simulink model "imugetmeas"  (R2025a)
settings: Solver=VariableStepAuto  StartTime=0.0  StopTime=10.0  RelTol=1e-3
undefined symbols (not defined in the file or in its folder): axang2rotm, fractalcoef
libraries: mspsensorlib x2
settings Model: Creator=nicolls  LastModifiedBy=nicolls

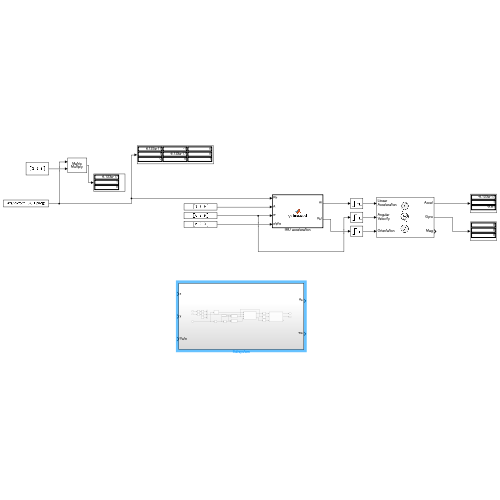
[thumbnail: Simulink's stored preview of the top-level diagram]
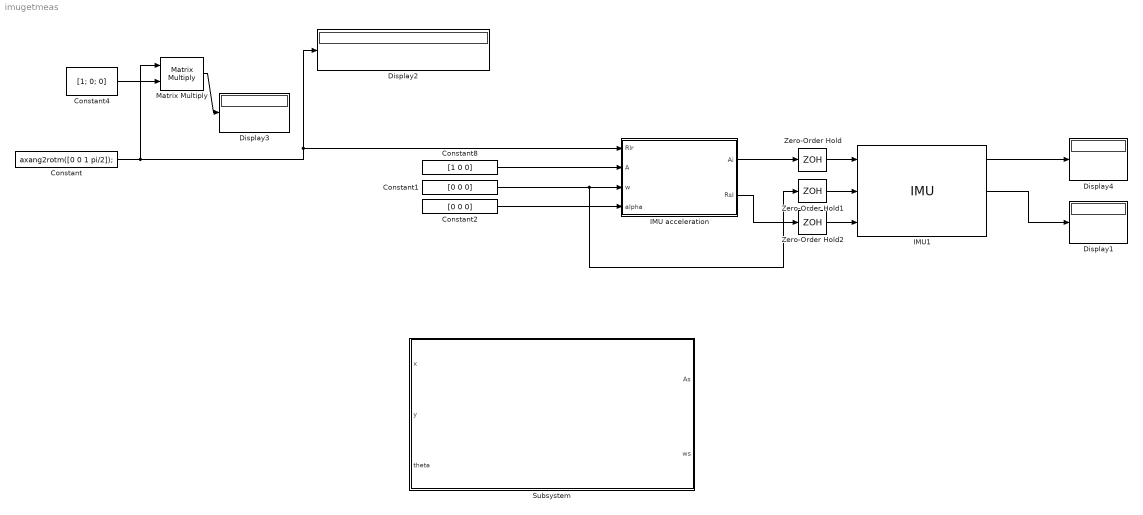
== system imugetmeas ==
  Constant : Constant  Value=axang2rotm([0 0 1 pi/2]);
  Constant1 : Constant  Value=[0 0 0]  VectorParams1D=off
  Constant2 : Constant  Value=[0 0 0]  VectorParams1D=off
  Constant4 : Constant  Value=[1; 0; 0]
  Constant8 : Constant  Value=[1 0 0]  VectorParams1D=off
  Display{1..4} (4 alike) : Display
  IMU acceleration : MATLAB Function  TreatAsAtomicUnit=on
  IMU1 : mspsensorlib/IMU  DispRefFrame=ENU  TemperaturePort=off  Temperature=25  MagneticFieldPort=off  MagneticFieldNED=[ 27.5550, -2.4169, -16.0849 ]  MagneticFieldENU=[ -2.4169, 27.5550, 16.0849 ]  SeedDouble=67  SimulateUsing=Interpreted execution  AccelParamsMeasurementRange=Inf  AccelParamsResolution=0  AccelParamsConstantBias=[ 0, 0, 0 ]  AccelParamsAxesMisalignment=[ 100, 0, 0; 0, 100, 0; 0, 0, 100 ]  AccelParamsNoiseDensity=[ 0, 0, 0 ]  AccelParamsBiasInstability=[ 0, 0, 0 ]  AccelParamsBiasInstabilityNumerator=fractalcoef().Numerator  AccelParamsBiasInstabilityDenominator=fractalcoef().Denominator  AccelParamsRandomWalk=[ 0, 0, 0 ]  AccelParamsNoiseType=double-sided  AccelParamsTemperatureBias=[ 0, 0, 0 ]  AccelParamsTemperatureScaleFactor=[ 0, 0, 0 ]  GyroParamsMeasurementRange=Inf  GyroParamsResolution=0  GyroParamsConstantBias=[ 0, 0, 0 ]  GyroParamsAxesMisalignment=[ 100, 0, 0; 0, 100, 0; 0, 0, 100 ]  GyroParamsAccelerationBias=[ 0, 0, 0 ]  GyroParamsNoiseDensity=[ 0, 0, 0 ]  GyroParamsBiasInstability=[ 0, 0, 0 ]  GyroParamsBiasInstabilityNumerator=fractalcoef().Numerator  GyroParamsBiasInstabilityDenominator=fractalcoef().Denominator  GyroParamsRandomWalk=[ 0, 0, 0 ]  GyroParamsNoiseType=double-sided  GyroParamsTemperatureBias=[ 0, 0, 0 ]  GyroParamsTemperatureScaleFactor=[ 0, 0, 0 ]  MagParamsMeasurementRange=Inf  MagParamsResolution=0  MagParamsConstantBias=[ 0, 0, 0 ]  MagParamsAxesMisalignment=[ 100, 0, 0; 0, 100, 0; 0, 0, 100 ]  MagParamsNoiseDensity=[ 0, 0, 0 ]  MagParamsBiasInstability=[ 0, 0, 0 ]  MagParamsBiasInstabilityNumerator=fractalcoef().Numerator  MagParamsBiasInstabilityDenominator=fractalcoef().Denominator  MagParamsRandomWalk=[ 0, 0, 0 ]  MagParamsNoiseType=double-sided  MagParamsTemperatureBias=[ 0, 0, 0 ]  MagParamsTemperatureScaleFactor=[ 0, 0, 0 ]
  Matrix Multiply : Product  Multiplication=Matrix(*)
  Subsystem : Subsystem
  Zero-Order Hold : ZeroOrderHold  SampleTime=0.02
  Zero-Order Hold1 : ZeroOrderHold  SampleTime=0.02
  Zero-Order Hold2 : ZeroOrderHold  SampleTime=0.02
  wires:
  Constant/1 -> Matrix Multiply/1, Display2/1, IMU acceleration/1(Rlr)
  Constant2/1 -> IMU acceleration/4(alpha)
  Matrix Multiply/1 -> Display3/1
  Constant4/1 -> Matrix Multiply/2
  IMU acceleration/1(Ai) -> Zero-Order Hold/1
  Constant1/1 -> Zero-Order Hold1/1, IMU acceleration/3(w)
  IMU1/1 -> Display4/1
  Zero-Order Hold/1 -> IMU1/1
  Zero-Order Hold1/1 -> IMU1/2
  Constant8/1 -> IMU acceleration/2(A)
  Zero-Order Hold2/1 -> IMU1/3
  IMU1/2 -> Display1/1
  IMU acceleration/2(Rsl) -> Zero-Order Hold2/1

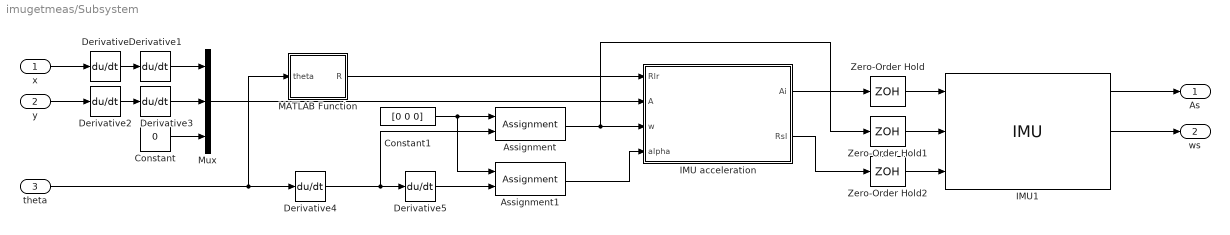
== system imugetmeas/Subsystem ==
  x : Inport
  y : Inport  Port=2
  theta : Inport  Port=3
  Assignment : Assignment  DiagnosticForDimensions=Warning  IndexOptions=Index vector (dialog)  Indices=3  OutputSizes=1
  Assignment1 : Assignment  DiagnosticForDimensions=Warning  IndexOptions=Index vector (dialog)  Indices=3  OutputSizes=1
  Constant : Constant  Value=0
  Constant1 : Constant  Value=[0 0 0]  VectorParams1D=off
  Derivative{,1..5} (6 alike) : Derivative
  IMU acceleration : MATLAB Function  TreatAsAtomicUnit=on
  IMU1 : mspsensorlib/IMU  DispRefFrame=ENU  TemperaturePort=off  Temperature=25  MagneticFieldPort=off  MagneticFieldNED=[ 27.5550, -2.4169, -16.0849 ]  MagneticFieldENU=[ -2.4169, 27.5550, 16.0849 ]  SeedDouble=67  SimulateUsing=Interpreted execution  AccelParamsMeasurementRange=Inf  AccelParamsResolution=0  AccelParamsConstantBias=[ 0, 0, 0 ]  AccelParamsAxesMisalignment=[ 100, 0, 0; 0, 100, 0; 0, 0, 100 ]  AccelParamsNoiseDensity=[ 0, 0, 0 ]  AccelParamsBiasInstability=[ 0, 0, 0 ]  AccelParamsBiasInstabilityNumerator=fractalcoef().Numerator  AccelParamsBiasInstabilityDenominator=fractalcoef().Denominator  AccelParamsRandomWalk=[ 0, 0, 0 ]  AccelParamsNoiseType=double-sided  AccelParamsTemperatureBias=[ 0, 0, 0 ]  AccelParamsTemperatureScaleFactor=[ 0, 0, 0 ]  GyroParamsMeasurementRange=Inf  GyroParamsResolution=0  GyroParamsConstantBias=[ 0, 0, 0 ]  GyroParamsAxesMisalignment=[ 100, 0, 0; 0, 100, 0; 0, 0, 100 ]  GyroParamsAccelerationBias=[ 0, 0, 0 ]  GyroParamsNoiseDensity=[ 0, 0, 0 ]  GyroParamsBiasInstability=[ 0, 0, 0 ]  GyroParamsBiasInstabilityNumerator=fractalcoef().Numerator  GyroParamsBiasInstabilityDenominator=fractalcoef().Denominator  GyroParamsRandomWalk=[ 0, 0, 0 ]  GyroParamsNoiseType=double-sided  GyroParamsTemperatureBias=[ 0, 0, 0 ]  GyroParamsTemperatureScaleFactor=[ 0, 0, 0 ]  MagParamsMeasurementRange=Inf  MagParamsResolution=0  MagParamsConstantBias=[ 0, 0, 0 ]  MagParamsAxesMisalignment=[ 100, 0, 0; 0, 100, 0; 0, 0, 100 ]  MagParamsNoiseDensity=[ 0, 0, 0 ]  MagParamsBiasInstability=[ 0, 0, 0 ]  MagParamsBiasInstabilityNumerator=fractalcoef().Numerator  MagParamsBiasInstabilityDenominator=fractalcoef().Denominator  MagParamsRandomWalk=[ 0, 0, 0 ]  MagParamsNoiseType=double-sided  MagParamsTemperatureBias=[ 0, 0, 0 ]  MagParamsTemperatureScaleFactor=[ 0, 0, 0 ]
  MATLAB Function : MATLAB Function  TreatAsAtomicUnit=on
  Mux : Mux  Inputs=3
  Zero-Order Hold : ZeroOrderHold  SampleTime=0.02
  Zero-Order Hold1 : ZeroOrderHold  SampleTime=0.02
  Zero-Order Hold2 : ZeroOrderHold  SampleTime=0.02
  As : Outport
  ws : Outport  Port=2
  wires:
  IMU acceleration/2(Rsl) -> Zero-Order Hold2/1
  Mux/1 -> IMU acceleration/2(A)
  IMU acceleration/1(Ai) -> Zero-Order Hold/1
  Zero-Order Hold/1 -> IMU1/1
  Zero-Order Hold1/1 -> IMU1/2
  IMU1/1 -> As/1
  Zero-Order Hold2/1 -> IMU1/3
  x/1 -> Derivative/1
  Derivative/1 -> Derivative1/1
  Derivative2/1 -> Derivative3/1
  y/1 -> Derivative2/1
  Derivative1/1 -> Mux/1
  Derivative3/1 -> Mux/2
  Constant/1 -> Mux/3
  IMU1/2 -> ws/1
  theta/1 -> MATLAB Function/1(theta), Derivative4/1
  MATLAB Function/1(R) -> IMU acceleration/1(Rlr)
  Constant1/1 -> Assignment1/1, Assignment/1
  Derivative4/1 -> Assignment/2, Derivative5/1
  Assignment/1 -> Zero-Order Hold1/1, IMU acceleration/3(w)
  Derivative5/1 -> Assignment1/2
  Assignment1/1 -> IMU acceleration/4(alpha)

== matlab function imugetmeas/Subsystem/IMU acceleration ==
  data: Ai output; Rsl output; Rlr input; A input; w input; alpha input; simstruct parameter
function [Ai,Rsl]  = getimuaccel(Rlr,A,w,alpha,simstruct)
%GETIMUACCEL  Get linear acceleration of IMU in local frame
%  [Ai,Rls]  = getimuaccel(Rlr,A,w,alpha,simstruct) calculates the linear
%  acceleration at the origin of an IMU sensor frame fixed to a robot.  The
%  robot frame is oriented by Rlr with respect to the local frane and is
%  moving according to (A,w,alpha) = (linear acceleration,angular
%  velocity,anglular acceleration). 
%
%  The function returns the linear acceleration As and the orientation Rsl
%  of the local frame in the sensor frame.  These two outputs are useful
%  for setting up the standard Simulink IMU block.

% Checks
if size(A,1)~=1 || size(A,2)~=3, error('Input A must be 1x3'); end
if size(w,1)~=1 || size(w,2)~=3, error('Input w must be 1x3'); end
if size(alpha,1)~=1 || size(alpha,2)~=3, error('Input alpha must be 1x3'); end

% Get sensor location vector (r_i-R) in local frame
si = Rlr*simstruct.timu;

% Kinematic equation (https://en.wikipedia.org/wiki/Rigid_body_dynamics,
% taking R as origin of robot frame).  This find the linear acceleration of
% the IMU in the local (inertial) navigation frame 
Ai = cross(alpha,si) + cross(w,cross(w,si)) + A;

% Get sensor orientation in local frame
Rrs = simstruct.Rimu;
Rls = Rlr*Rrs;
Rsl = inv(Rls);

% Generate measurements in sensor frame
Ait = Ai;  Ait(3) = Ait(3) + 9.81;  % add gravity
As = (inv(Rls)*Ait')';  
ws = (inv(Rls)*w')';

== matlab function imugetmeas/IMU acceleration ==
  data: Ai output; Rsl output; Rlr input; A input; w input; alpha input; simstruct parameter
function [Ai,Rsl]  = getimuaccel(Rlr,A,w,alpha,simstruct)
%GETIMUACCEL  Get linear acceleration of IMU in local frame
%  [Ai,Rls]  = getimuaccel(Rlr,A,w,alpha,simstruct) calculates the linear
%  acceleration at the origin of an IMU sensor frame fixed to a robot.  The
%  robot frame is oriented by Rlr with respect to the local frane and is
%  moving according to (A,w,alpha) = (linear acceleration,angular
%  velocity,anglular acceleration). 
%
%  The function returns the linear acceleration As and the orientation Rsl
%  of the local frame in the sensor frame.  These two outputs are useful
%  for setting up the standard Simulink IMU block.

% Checks
if size(A,1)~=1 || size(A,2)~=3, error('Input A must be 1x3'); end
if size(w,1)~=1 || size(w,2)~=3, error('Input w must be 1x3'); end
if size(alpha,1)~=1 || size(alpha,2)~=3, error('Input alpha must be 1x3'); end

% Get sensor location vector (r_i-R) in local frame
si = Rlr*simstruct.timu;

% Kinematic equation (https://en.wikipedia.org/wiki/Rigid_body_dynamics,
% taking R as origin of robot frame).  This find the linear acceleration of
% the IMU in the local (inertial) navigation frame 
Ai = cross(alpha,si) + cross(w,cross(w,si)) + A;

% Get sensor orientation in local frame
Rrs = simstruct.Rimu;
Rls = Rlr*Rrs;
Rsl = inv(Rls);

% Generate measurements in sensor frame
Ait = Ai;  Ait(3) = Ait(3) + 9.81;  % add gravity
As = (inv(Rls)*Ait')';  
ws = (inv(Rls)*w')';

== matlab function imugetmeas/Subsystem/MATLAB Function ==
  data: theta input; R output
function R = theta2R(theta)

R = axang2rotm([0 0 1 theta]);
